simulink model "CtrlStrct_VNT_Level1"  (R2018a)
settings: Solver=VariableStepAuto  StartTime=0.0  StopTime=10  FixedStep=sampletime  RelTol=1e-3  EnableMultiTasking=on
PreLoadFcn:
  | CtrlStrct_SmplCAN_BusInfo
libraries: canmsglib x56, simulink x1
(part 1 of 3)
settings Model: Creator=IAEC nishito  LastModifiedBy=E00026
settings DataIOCC: LimitDataPoints=on  SaveFormat=Array  SaveOutput=off  SaveTime=off
settings OptimizationCC: DefaultParameterBehavior=Inlined  ExpressionDepthLimit=2147483647  LifeSpan=inf
settings DebuggingCC: UnderspecifiedInitializationDetection=Classic  MergeDetectMultiDrivingBlocksExec=none  SolverPrmCheckMsg=warning  InheritedTsInSrcMsg=none  FcnCallInpInsideContextMsg=warning  StateNameClashWarn=warning  SFUnexpectedBacktrackingDiag=warning  SFNoUnconditionalDefaultTransitionDiag=warning  SFExecutionAtInitializationDiag=none
settings HardwareCC: ProdBitPerPointer=32  ProdBitPerSizeT=32  ProdBitPerPtrDiffT=32  ProdLargestAtomicFloat=None  ProdIntDivRoundTo=Undefined  ProdEndianess=Unspecified  ProdWordSize=32  ProdHWDeviceType=32-bit Generic
settings ModelReferenceCC: ModelReferenceNumInstancesAllowed=Single  PropagateSignalLabelsOutOfModel=off
settings CodeAppCC: StateflowObjectComments=on
settings GRTTargetCC: TargetLangStandard=C89/C90 (ANSI)  GeneratePreprocessorConditionals=Disable all  CombineOutputUpdateFcns=off  GRTInterface=on
settings ConfigComp: CovMetricSettings=dw  CovHtmlReporting=on  CovSaveCumulativeToWorkspaceVar=on  CovSaveSingleToWorkspaceVar=on  CovExternalEMLEnable=off

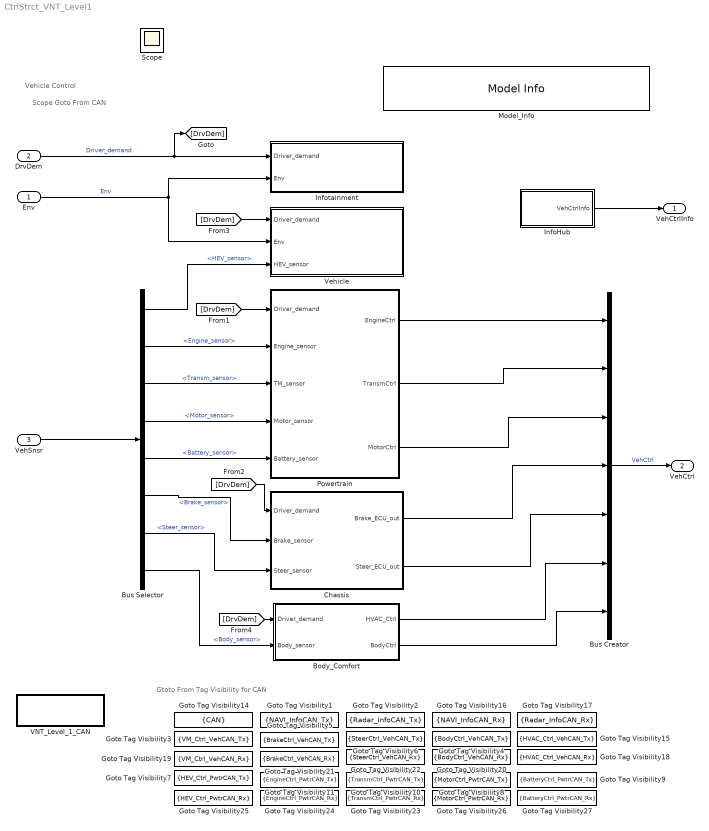
== system CtrlStrct_VNT_Level1 ==
  note: Scope Goto From CAN
  note: Gtoto From Tag Visibility for CAN
  note: Vehicle Control
  Env : Inport  OutDataTypeStr=Bus: Environment_Bus
      settings: AttributesFormatString=<%<OutDataTypeStr>>
  DrvDem : Inport  Port=2  OutDataTypeStr=Bus: Driver_demand_Bus
      settings: AttributesFormatString=%<OutDataTypeStr>
  VehSnsr : Inport  Port=3  OutDataTypeStr=Bus: Vehicle_sensor_Bus
      settings: AttributesFormatString=<%<OutDataTypeStr>>
  Body_Comfort : Subsystem
  Bus Creator : BusCreator  Inputs=7  OutDataTypeStr=Bus: Ctrl_intg_Bus
      settings: AttributesFormatString=%<OutDataTypeStr>
  Bus Selector : BusSelector  OutputSignals=HEV_sensor,Engine_sensor,Transm_sensor,Motor_sensor,Battery_sensor,Brake_sensor,Steer_sensor,Body_sensor
  Chassis : Subsystem
  Goto Tag Visibility1 : GotoTagVisibility  GotoTag=NAVI_InfoCAN_Tx
  Goto Tag Visibility10 : GotoTagVisibility  GotoTag=TransmCtrl_PwtrCAN_Tx
  Goto Tag Visibility11 : GotoTagVisibility  GotoTag=EngineCtrl_PwtrCAN_Tx
  Goto Tag Visibility14 : GotoTagVisibility  GotoTag=CAN
  Goto Tag Visibility15 : GotoTagVisibility  GotoTag=HVAC_Ctrl_VehCAN_Tx
  Goto Tag Visibility16 : GotoTagVisibility  GotoTag=NAVI_InfoCAN_Rx
  Goto Tag Visibility17 : GotoTagVisibility  GotoTag=Radar_InfoCAN_Rx
  Goto Tag Visibility18 : GotoTagVisibility  GotoTag=HVAC_Ctrl_VehCAN_Rx
  Goto Tag Visibility19 : GotoTagVisibility  GotoTag=VM_Ctrl_VehCAN_Rx
  Goto Tag Visibility2 : GotoTagVisibility  GotoTag=Radar_InfoCAN_Tx
  Goto Tag Visibility20 : GotoTagVisibility  GotoTag=BodyCtrl_VehCAN_Rx
  Goto Tag Visibility21 : GotoTagVisibility  GotoTag=BrakeCtrl_VehCAN_Rx
  Goto Tag Visibility22 : GotoTagVisibility  GotoTag=SteerCtrl_VehCAN_Rx
  Goto Tag Visibility23 : GotoTagVisibility  GotoTag=TransmCtrl_PwtrCAN_Rx
  Goto Tag Visibility24 : GotoTagVisibility  GotoTag=EngineCtrl_PwtrCAN_Rx
  Goto Tag Visibility25 : GotoTagVisibility  GotoTag=HEV_Ctrl_PwtrCAN_Rx
  Goto Tag Visibility26 : GotoTagVisibility  GotoTag=MotorCtrl_PwtrCAN_Rx
  Goto Tag Visibility27 : GotoTagVisibility  GotoTag=BatteryCtrl_PwtrCAN_Rx
  Goto Tag Visibility3 : GotoTagVisibility  GotoTag=VM_Ctrl_VehCAN_Tx
  Goto Tag Visibility4 : GotoTagVisibility  GotoTag=BodyCtrl_VehCAN_Tx
  Goto Tag Visibility5 : GotoTagVisibility  GotoTag=BrakeCtrl_VehCAN_Tx
  Goto Tag Visibility6 : GotoTagVisibility  GotoTag=SteerCtrl_VehCAN_Tx
  Goto Tag Visibility7 : GotoTagVisibility  GotoTag=HEV_Ctrl_PwtrCAN_Tx
  Goto Tag Visibility8 : GotoTagVisibility  GotoTag=MotorCtrl_PwtrCAN_Tx
  Goto Tag Visibility9 : GotoTagVisibility  GotoTag=BatteryCtrl_PwtrCAN_Tx
  InfoHub : Subsystem
  Infotainment : Subsystem
  Model_Info : simulink/Model-Wide Utilities/Model Info  Frame=on  DisplayStringWithTags=|  HorizontalTextAlignment=Left  LeftAlignmentValue=0.02
      | Version  %<ModelVersion>
      | LastModifided by %<LastModifiedBy>  Date %<LastModificationDate>
      | Description  %<Description>
  Powertrain : Subsystem
  VNT_Level_1_CAN : Subsystem  VariantControl=VarObj_CanType_VNT_simu
  Vehicle : Subsystem
  VehCtrlInfo : Outport  OutDataTypeStr=Bus: IntgCtrl_Info_Bus
      settings: AttributesFormatString=<%<OutDataTypeStr>>
  VehCtrl : Outport  Port=2  OutDataTypeStr=Bus: Ctrl_intg_Bus
      settings: AttributesFormatString=<%<OutDataTypeStr>>
  Scope : Scope
  wires:
  InfoHub/1(VehCtrlInfo) -> VehCtrlInfo/1
  Chassis/2(Steer_ECU_out) -> Bus Creator/5
  Env/1 -> Vehicle/2(Env), Infotainment/2(Env)  "Env"
  Bus Creator/1 -> VehCtrl/1  "VehCtrl"
  [DrvDem] -> Powertrain/1(Driver_demand)
  Powertrain/3(MotorCtrl) -> Bus Creator/3
  Bus Selector/3 -> Powertrain/3(TM_sensor)  "<Transm_sensor>"
  Bus Selector/6 -> Chassis/2(Brake_sensor)  "<Brake_sensor>"
  Body_Comfort/2(BodyCtrl) -> Bus Creator/7
  Bus Selector/2 -> Powertrain/2(Engine_sensor)  "<Engine_sensor>"
  Powertrain/2(TransmCtrl) -> Bus Creator/2
  Chassis/1(Brake_ECU_out) -> Bus Creator/4
  VehSnsr/1 -> Bus Selector/1
  [DrvDem] -> Chassis/1(Driver_demand)
  Body_Comfort/1(HVAC_Ctrl) -> Bus Creator/6
  Bus Selector/1 -> Vehicle/3(HEV_sensor)  "<HEV_sensor>"
  Bus Selector/7 -> Chassis/3(Steer_sensor)  "<Steer_sensor>"
  Powertrain/1(EngineCtrl) -> Bus Creator/1
  [DrvDem] -> Vehicle/1(Driver_demand)
  Bus Selector/5 -> Powertrain/5(Battery_sensor)  "<Battery_sensor>"
  DrvDem/1 -> [DrvDem], Infotainment/1(Driver_demand)  "Driver_demand"
  Bus Selector/8 -> Body_Comfort/2(Body_sensor)  "<Body_sensor>"
  Bus Selector/4 -> Powertrain/4(Motor_sensor)  "<Motor_sensor>"
  [DrvDem] -> Body_Comfort/1(Driver_demand)

== system CtrlStrct_VNT_Level1/Body_Comfort ==
  note: Body Control
  Driver_demand : Inport
  Body_sensor : Inport  Port=2
  Body_Control : Subsystem
  HVAC_Control : Subsystem
  HVAC_Ctrl : Outport
  BodyCtrl : Outport  Port=2
  wires:
  Body_Control/1(BodyCtrl) -> BodyCtrl/1
  Driver_demand/1 -> HVAC_Control/1(Driver_demand), Body_Control/1(Driver_demand)
  Body_sensor/1 -> HVAC_Control/2(Body_sensor), Body_Control/2(Body_sensor)
  HVAC_Control/1(HVAC_Ctrl) -> HVAC_Ctrl/1

== system CtrlStrct_VNT_Level1/Chassis ==
  note: Chassis Control
  Driver_demand : Inport
  Brake_sensor : Inport  Port=2
  Steer_sensor : Inport  Port=3
  Brake_Control : Subsystem
  Steer_Control : Subsystem
  Brake_ECU_out : Outport
  Steer_ECU_out : Outport  Port=2
  wires:
  Driver_demand/1 -> Brake_Control/1(Driver_demand), Steer_Control/1(Driver_demand)
  Brake_Control/1(BrakeCtrl) -> Brake_ECU_out/1
  Brake_sensor/1 -> Brake_Control/2(Brake_sensor)
  Steer_Control/1(SteerCtrl) -> Steer_ECU_out/1
  Steer_sensor/1 -> Steer_Control/2(Steer_sensor)

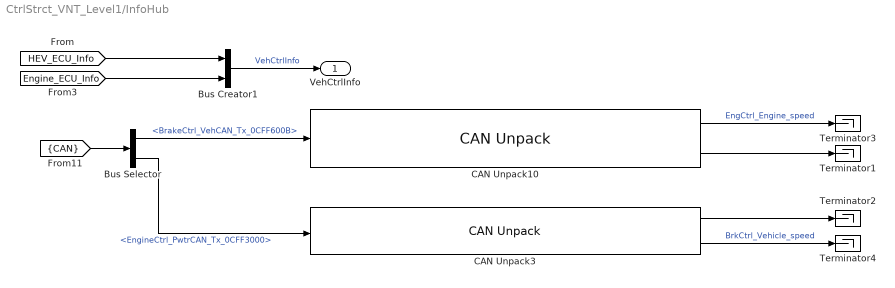
== system CtrlStrct_VNT_Level1/InfoHub ==
  Bus Creator1 : BusCreator  Inputs=2
  Bus Selector : BusSelector  OutputSignals=VehCAN.BrakeCtrl_VehCAN_Tx_0CFF600B,PwtrCAN.EngineCtrl_PwtrCAN_Tx_0CFF3000
  CAN Unpack10 : canmsglib/CAN Unpack  CANdbFile=C:\Users\aa781680\OneDrive - YanmarGlobal\MainStrage\04_MATLAB\JMAAB_CoopCon\CoopConModel\20180726_18a_ymr\Project\CANDB\HEV_CANDB.dbc  MsgList=EngineCtrl_PwtrCAN_Tx  MsgName=EngineCtrl_PwtrCAN_Tx  MsgIDType=Extended (29-bit identifier)  MsgIdentifier=218050560  MsgLength=8  SignalInfo=EngCtrl_Engine_speed$0$16$1$2$1$0$1.250000e-01$0$0$8192$#EngCtrl_Engine_torque_actual$16$16$1$1$1$0$1.562500e-02$0$-300$300$#  NSignals=2  IDPort=off  TimestampPort=off  ErrorPort=off  RemotePort=off  LengthPort=off  StatusPort=off  StartBits=str2num('[int32(0);int32(16)]')  SignalSizes=str2num('[int32(16);int32(16)]')  ByteOrders=str2num('[int32(1);int32(1)]')  DataTypes=str2num('[int32(2);int32(1)]')  MultiplexTypes=str2num('[int32(1);int32(1)]')  MultiplexValues=str2num('[double(0);double(0)]')  Factors=str2num('[double(1.250000e-01);double(1.562500e-02)]')  Offsets=str2num('[double(0);double(0)]')  Minimums=str2num('[double(0);double(-300)]')  Maximums=str2num('[double(8192);double(300)]')  ApplyMinMax=off
      settings: SourceProductName=Simulink Real-Time  SourceProductBaseCode=XP  DataFormat=CANdb specified signals
  CAN Unpack3 : canmsglib/CAN Unpack  CANdbFile=C:\Users\aa781680\OneDrive - YanmarGlobal\MainStrage\04_MATLAB\JMAAB_CoopCon\CoopConModel\20180726_18a_ymr\Project\CANDB\HEV_CANDB.dbc  MsgList=BrakeCtrl_VehCAN_Tx  MsgName=BrakeCtrl_VehCAN_Tx  MsgIDType=Extended (29-bit identifier)  MsgIdentifier=218062859  MsgLength=8  SignalInfo=BrkCtrl_Regen_brake_torque_reque$16$16$1$1$1$0$1.000000e-02$0$-300$300$#BrkCtrl_Vehicle_speed$0$16$1$2$1$0$1.000000e-01$0$0$180$#  NSignals=2  IDPort=off  TimestampPort=off  ErrorPort=off  RemotePort=off  LengthPort=off  StatusPort=off  StartBits=str2num('[int32(16);int32(0)]')  SignalSizes=str2num('[int32(16);int32(16)]')  ByteOrders=str2num('[int32(1);int32(1)]')  DataTypes=str2num('[int32(1);int32(2)]')  MultiplexTypes=str2num('[int32(1);int32(1)]')  MultiplexValues=str2num('[double(0);double(0)]')  Factors=str2num('[double(1.000000e-02);double(1.000000e-01)]')  Offsets=str2num('[double(0);double(0)]')  Minimums=str2num('[double(-300);double(0)]')  Maximums=str2num('[double(300);double(180)]')  ApplyMinMax=off
      settings: SourceProductName=Simulink Real-Time  SourceProductBaseCode=XP  DataFormat=CANdb specified signals
  Terminator{1..4} (4 alike) : Terminator
  VehCtrlInfo : Outport
  wires:
  [CAN] -> Bus Selector/1
  Bus Creator1/1 -> VehCtrlInfo/1  "VehCtrlInfo"
  [Engine_ECU_Info] -> Bus Creator1/2
  [HEV_ECU_Info] -> Bus Creator1/1
  CAN Unpack10/2 -> Terminator1/1
  CAN Unpack3/1 -> Terminator2/1
  Bus Selector/1 -> CAN Unpack10/1  "<BrakeCtrl_VehCAN_Tx_0CFF600B>"
  Bus Selector/2 -> CAN Unpack3/1  "<EngineCtrl_PwtrCAN_Tx_0CFF3000>"
  CAN Unpack10/1 -> Terminator3/1  "EngCtrl_Engine_speed"
  CAN Unpack3/2 -> Terminator4/1  "BrkCtrl_Vehicle_speed"

== system CtrlStrct_VNT_Level1/Infotainment ==
  note: Infotainment
  Driver_demand : Inport
  Env : Inport  Port=2
  Navigation : Subsystem
  Radar_Detection : Subsystem
  wires:
  Env/1 -> Navigation/2(Env), Radar_Detection/2(Env)
  Driver_demand/1 -> Radar_Detection/1(Driver_demand), Navigation/1(Driver_demand)

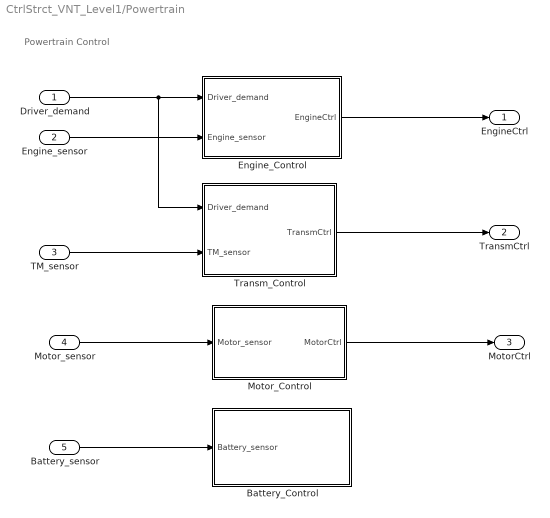
== system CtrlStrct_VNT_Level1/Powertrain ==
  note: Powertrain Control
  Driver_demand : Inport
  Engine_sensor : Inport  Port=2
  TM_sensor : Inport  Port=3
  Motor_sensor : Inport  Port=4
  Battery_sensor : Inport  Port=5
  Battery_Control : Subsystem
  Engine_Control : Subsystem
  Motor_Control : Subsystem
  Transm_Control : Subsystem
  EngineCtrl : Outport
  TransmCtrl : Outport  Port=2
  MotorCtrl : Outport  Port=3
  wires:
  Driver_demand/1 -> Transm_Control/1(Driver_demand), Engine_Control/1(Driver_demand)
  Motor_Control/1(MotorCtrl) -> MotorCtrl/1
  Motor_sensor/1 -> Motor_Control/1(Motor_sensor)
  Battery_sensor/1 -> Battery_Control/1(Battery_sensor)
  Engine_Control/1(EngineCtrl) -> EngineCtrl/1
  Engine_sensor/1 -> Engine_Control/2(Engine_sensor)
  Transm_Control/1(TransmCtrl) -> TransmCtrl/1
  TM_sensor/1 -> Transm_Control/2(TM_sensor)

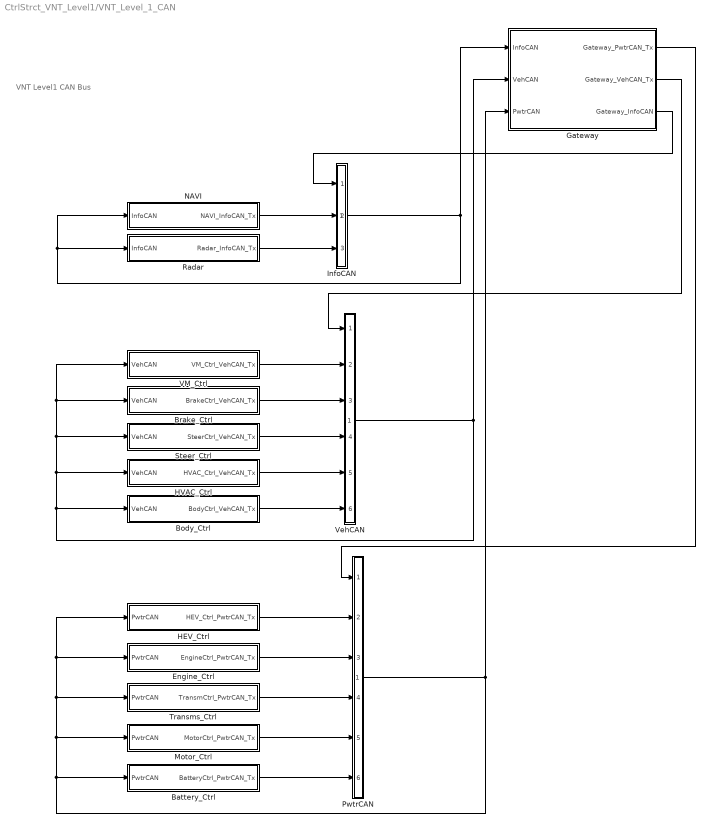
== system CtrlStrct_VNT_Level1/VNT_Level_1_CAN ==
  note: VNT Level1 CAN Bus
  Battery_Ctrl : Subsystem
  Body_Ctrl : Subsystem
  Brake_Ctrl : Subsystem
  Engine_Ctrl : Subsystem
  Gateway : Subsystem
  HEV_Ctrl : Subsystem
  HVAC_Ctrl : Subsystem
  InfoCAN : Subsystem
  Motor_Ctrl : Subsystem
  NAVI : Subsystem
  PwtrCAN : Subsystem
  Radar : Subsystem
  Steer_Ctrl : Subsystem
  Transms_Ctrl : Subsystem
  VM_Ctrl : Subsystem
  VehCAN : Subsystem
  wires:
  PwtrCAN/1(PwtrCAN) -> Battery_Ctrl/1(PwtrCAN), Motor_Ctrl/1(PwtrCAN), Transms_Ctrl/1(PwtrCAN), Engine_Ctrl/1(PwtrCAN), HEV_Ctrl/1(PwtrCAN), Gateway/3(PwtrCAN)
  Gateway/1(Gateway_PwtrCAN_Tx) -> PwtrCAN/1(Gateway_PwtrCAN_Tx)
  HEV_Ctrl/1(HEV_Ctrl_PwtrCAN_Tx) -> PwtrCAN/2(HEV_Ctrl_PwtrCAN_Tx)
  Engine_Ctrl/1(EngineCtrl_PwtrCAN_Tx) -> PwtrCAN/3(EngineCtrl_PwtrCAN_Tx)
  Transms_Ctrl/1(TransmCtrl_PwtrCAN_Tx) -> PwtrCAN/4(TransmCtrl_PwtrCAN_Tx)
  Motor_Ctrl/1(MotorCtrl_PwtrCAN_Tx) -> PwtrCAN/5(MotorCtrl_PwtrCAN_Tx)
  Battery_Ctrl/1(BatteryCtrl_PwtrCAN_Tx) -> PwtrCAN/6(BatteryCtrl_PwtrCAN_Tx)
  VehCAN/1(VehCAN) -> Body_Ctrl/1(VehCAN), HVAC_Ctrl/1(VehCAN), Steer_Ctrl/1(VehCAN), Brake_Ctrl/1(VehCAN), VM_Ctrl/1(VehCAN), Gateway/2(VehCAN)
  Gateway/2(Gateway_VehCAN_Tx) -> VehCAN/1(Gateway_VehCAN_Tx)
  VM_Ctrl/1(VM_Ctrl_VehCAN_Tx) -> VehCAN/2(VM_Ctrl_VehCAN_Tx)
  Brake_Ctrl/1(BrakeCtrl_VehCAN_Tx) -> VehCAN/3(BrakeCtrl_VehCAN_Tx)
  Steer_Ctrl/1(SteerCtrl_VehCAN_Tx) -> VehCAN/4(SteerCtrl_VehCAN_Tx)
  HVAC_Ctrl/1(HVAC_Ctrl_VehCAN_Tx) -> VehCAN/5(HVAC_Ctrl_VehCAN_Tx)
  Body_Ctrl/1(BodyCtrl_VehCAN_Tx) -> VehCAN/6(BodyCtrl_VehCAN_Tx)
  InfoCAN/1(InfoCAN) -> Radar/1(InfoCAN), NAVI/1(InfoCAN), Gateway/1(InfoCAN)
  Gateway/3(Gateway_InfoCAN) -> InfoCAN/1(Gateway_InfoCAN)
  NAVI/1(NAVI_InfoCAN_Tx) -> InfoCAN/2(NAVI_InfoCAN_Tx)
  Radar/1(Radar_InfoCAN_Tx) -> InfoCAN/3(Radar_InfoCAN_Tx)

== system CtrlStrct_VNT_Level1/Vehicle ==
  note: Vehicle Integrated Control
  Driver_demand : Inport
  Env : Inport  Port=2
  HEV_sensor : Inport  Port=3
  HEV_Control : Subsystem
  Vehicle_Motion_Control : Subsystem
  wires:
  Env/1 -> Vehicle_Motion_Control/1(Env)
  Driver_demand/1 -> HEV_Control/1(Driver_demand)
  HEV_sensor/1 -> HEV_Control/2(HEV_sensor)

== system CtrlStrct_VNT_Level1/Body_Comfort/Body_Control ==
  note: Body Control
  Driver_demand : Inport
  Body_sensor : Inport  Port=2
  BodyControlModule : ModelReference  ModelNameDialog=BodyCtrl_V1_1.slx  ModelReferenceVersion=0.1.16
  Rate Transition1 : RateTransition  Deterministic=off
      settings: AttributesFormatString=<Deterministic=%<Deterministic>>
  Rate Transition2 : RateTransition  Deterministic=off
      settings: AttributesFormatString=<Deterministic=%<Deterministic>>
  Rate Transition4 : RateTransition  Deterministic=off
      settings: AttributesFormatString=<Deterministic=%<Deterministic>>
  BodyCtrl : Outport
  tag scope: BodyCtrl_VehCAN_Tx=scoped
  wires:
  Driver_demand/1 -> Rate Transition2/1
  Rate Transition2/1 -> BodyControlModule/1
  BodyControlModule/1 -> Rate Transition4/1
  [BodyCtrl_VehCAN_Rx] -> BodyControlModule/3
  BodyControlModule/2 -> [BodyCtrl_VehCAN_Tx]  "BodyCtrl_VehCAN_Tx"
  Rate Transition4/1 -> BodyCtrl/1  "BodyCtrl"
  Body_sensor/1 -> Rate Transition1/1
  Rate Transition1/1 -> BodyControlModule/2

== system CtrlStrct_VNT_Level1/Body_Comfort/HVAC_Control ==
  note: HVAC Control
  Driver_demand : Inport
  Body_sensor : Inport  Port=2
  Aircon_Control : ModelReference  ModelNameDialog=HVAC_Ctrl_V1_1.slx  ModelReferenceVersion=0.1.25
  Rate Transition1 : RateTransition  Deterministic=off
      settings: AttributesFormatString=<Deterministic=%<Deterministic>>
  Rate Transition2 : RateTransition  Deterministic=off
      settings: AttributesFormatString=<Deterministic=%<Deterministic>>
  Rate Transition4 : RateTransition  Deterministic=off
      settings: AttributesFormatString=<Deterministic=%<Deterministic>>
  HVAC_Ctrl : Outport
  tag scope: HVAC_Ctrl_VehCAN_Tx=scoped
  wires:
  Rate Transition1/1 -> Aircon_Control/2
  Body_sensor/1 -> Rate Transition1/1
  Rate Transition4/1 -> HVAC_Ctrl/1  "HVAC_Ctrl"
  Aircon_Control/2 -> [HVAC_Ctrl_VehCAN_Tx]  "HVAC_Ctrl_VehCAN_Tx"
  [HVAC_Ctrl_VehCAN_Rx] -> Aircon_Control/3
  Aircon_Control/1 -> Rate Transition4/1
  Rate Transition2/1 -> Aircon_Control/1
  Driver_demand/1 -> Rate Transition2/1

== system CtrlStrct_VNT_Level1/Chassis/Brake_Control ==
  note: Brake Control
  Driver_demand : Inport
  Brake_sensor : Inport  Port=2
  Brake_Control : ModelReference  ModelNameDialog=BrakeCtrl_V1_1.slx  ModelReferenceVersion=1.0.23
  Rate Transition1 : RateTransition  Deterministic=off
      settings: AttributesFormatString=<Deterministic=%<Deterministic>>
  Rate Transition2 : RateTransition  Deterministic=off
      settings: AttributesFormatString=<Deterministic=%<Deterministic>>
  Rate Transition4 : RateTransition  Deterministic=off
      settings: AttributesFormatString=<Deterministic=%<Deterministic>>
  Terminator : Terminator
  BrakeCtrl : Outport
  tag scope: BrakeCtrl_VehCAN_Tx=scoped
  wires:
  Rate Transition2/1 -> Brake_Control/2
  Driver_demand/1 -> Rate Transition1/1
  Rate Transition1/1 -> Brake_Control/1
  Brake_sensor/1 -> Rate Transition2/1
  Brake_Control/3 -> Terminator/1
  [BrakeCtrl_VehCAN_Rx] -> Brake_Control/3
  Rate Transition4/1 -> BrakeCtrl/1  "BrakeCtrl"
  Brake_Control/1 -> Rate Transition4/1
  Brake_Control/2 -> [BrakeCtrl_VehCAN_Tx]  "BrakeCtrl_VehCAN_Tx"

== system CtrlStrct_VNT_Level1/Chassis/Steer_Control ==
  note: Steering Control
  Driver_demand : Inport
  Steer_sensor : Inport  Port=2
  Rate Transition3 : RateTransition  Deterministic=off
      settings: AttributesFormatString=<Deterministic=%<Deterministic>>
  Rate Transition4 : RateTransition  Deterministic=off
      settings: AttributesFormatString=<Deterministic=%<Deterministic>>
  Rate Transition5 : RateTransition  Deterministic=off
      settings: AttributesFormatString=<Deterministic=%<Deterministic>>
  Steer_Control : ModelReference  ModelNameDialog=SteerCtrl_V1_1.slx  ModelReferenceVersion=0.1.16
  SteerCtrl : Outport
  tag scope: SteerCtrl_VehCAN_Tx=scoped
  wires:
  Rate Transition4/1 -> Steer_Control/2
  Driver_demand/1 -> Rate Transition3/1
  Steer_Control/1 -> Rate Transition5/1
  Steer_sensor/1 -> Rate Transition4/1
  [SteerCtrl_VehCAN_Rx] -> Steer_Control/3
  Rate Transition3/1 -> Steer_Control/1
  Rate Transition5/1 -> SteerCtrl/1  "SteerCtrl"
  Steer_Control/2 -> [SteerCtrl_VehCAN_Tx]  "SteerCtrl_VehCAN_Tx"

== system CtrlStrct_VNT_Level1/Infotainment/Navigation ==
  note: Navigation
  Driver_demand : Inport
  Env : Inport  Port=2
  NAVI : ModelReference  ModelNameDialog=NAVI_V1_1.slx  ModelReferenceVersion=0.1.17
  Rate Transition1 : RateTransition  Deterministic=off
      settings: AttributesFormatString=<Deterministic=%<Deterministic>>
  Rate Transition4 : RateTransition  Deterministic=off
      settings: AttributesFormatString=<Deterministic=%<Deterministic>>
  tag scope: NAVI_InfoCAN_Tx=scoped
  wires:
  Rate Transition1/1 -> NAVI/1
  Driver_demand/1 -> Rate Transition1/1
  [NAVI_InfoCAN_Rx] -> NAVI/3
  NAVI/1 -> [NAVI_InfoCAN_Tx]  "NAVI_InfoCAN_Tx"
  Env/1 -> Rate Transition4/1
  Rate Transition4/1 -> NAVI/2

== system CtrlStrct_VNT_Level1/Infotainment/Radar_Detection ==
  note: Radar Detection
  Driver_demand : Inport
  Env : Inport  Port=2
  Radar_Detection : ModelReference  ModelNameDialog=Radar_V1_1.slx  ModelReferenceVersion=0.1.17
  Rate Transition1 : RateTransition  Deterministic=off
      settings: AttributesFormatString=<Deterministic=%<Deterministic>>
  Rate Transition4 : RateTransition  Deterministic=off
      settings: AttributesFormatString=<Deterministic=%<Deterministic>>
  tag scope: Radar_InfoCAN_Tx=scoped
  wires:
  Rate Transition1/1 -> Radar_Detection/2
  Env/1 -> Rate Transition1/1
  [Radar_InfoCAN_Rx] -> Radar_Detection/3
  Radar_Detection/1 -> [Radar_InfoCAN_Tx]  "Radar_InfoCAN_Tx"
  Driver_demand/1 -> Rate Transition4/1
  Rate Transition4/1 -> Radar_Detection/1

== system CtrlStrct_VNT_Level1/Powertrain/Battery_Control ==
  note: Battery Control
  Battery_sensor : Inport
  Battery_Control : ModelReference  ModelNameDialog=BatteryCtrl_V1_1.slx  ModelReferenceVersion=0.1.22
  Rate Transition1 : RateTransition  Deterministic=off
      settings: AttributesFormatString=<Deterministic=%<Deterministic>>
  tag scope: BatteryCtrl_PwtrCAN_Tx=scoped
  wires:
  Battery_sensor/1 -> Rate Transition1/1
  [BatteryCtrl_PwtrCAN_Rx] -> Battery_Control/2
  Rate Transition1/1 -> Battery_Control/1
  Battery_Control/1 -> [BatteryCtrl_PwtrCAN_Tx]  "BatteryCtrl_PwtrCAN_Tx"

== system CtrlStrct_VNT_Level1/Powertrain/Engine_Control ==
  note: Engine Control
  Driver_demand : Inport
  Engine_sensor : Inport  Port=2
  Engine_Control : Subsystem  Variant=on
  Info_in : Subsystem
  Rate Transition{1..2,5..6} (4 alike) : RateTransition  Deterministic=off
      settings: AttributesFormatString=<Deterministic=%<Deterministic>>
  EngineCtrl : Outport
  tag scope: EngineCtrl_PwtrCAN_Tx=scoped, Engine_ECU_Info=global
  wires:
  Driver_demand/1 -> Rate Transition1/1
  Engine_sensor/1 -> Rate Transition2/1
  Rate Transition5/1 -> EngineCtrl/1  "EngineCtrl"
  Rate Transition6/1 -> [Engine_ECU_Info]  "EngineCtrl_Info"
  Engine_Control/2(" EngineCtrl_PwtrCAN_Tx") -> [EngineCtrl_PwtrCAN_Tx]  "EngineCtrl_PwtrCAN_Tx"
  Rate Transition1/1 -> Engine_Control/1("DrvDem ")
  Rate Transition2/1 -> Engine_Control/2("Eng_Sns ")
  [EngineCtrl_PwtrCAN_Rx] -> Engine_Control/3(EngineCtrl_PwtrCAN_Rx)
  Info_in/1(Info_in) -> Engine_Control/4("Info_in ")
  Engine_Control/1(" EngineCtrl") -> Rate Transition5/1
  Engine_Control/3(" EngineCtrl_Info") -> Rate Transition6/1

== system CtrlStrct_VNT_Level1/Powertrain/Motor_Control ==
  note: Motor Control
  Motor_sensor : Inport
  Motor_Control : ModelReference  ModelNameDialog=MotorCtrl_V1_1.slx  ModelReferenceVersion=1.0.21
  Rate Transition1 : RateTransition  Deterministic=off
      settings: AttributesFormatString=<Deterministic=%<Deterministic>>
  Rate Transition3 : RateTransition  Deterministic=off
      settings: AttributesFormatString=<Deterministic=%<Deterministic>>
  Terminator : Terminator
  MotorCtrl : Outport
  tag scope: MotorCtrl_PwtrCAN_Tx=scoped
  wires:
  Rate Transition1/1 -> Motor_Control/1
  [MotorCtrl_PwtrCAN_Rx] -> Motor_Control/2
  Motor_sensor/1 -> Rate Transition1/1
  Motor_Control/3 -> Terminator/1
  Rate Transition3/1 -> MotorCtrl/1  "MotorCtrl"
  Motor_Control/1 -> Rate Transition3/1
  Motor_Control/2 -> [MotorCtrl_PwtrCAN_Tx]  "MotorCtrl_PwtrCAN_Tx"

== system CtrlStrct_VNT_Level1/Powertrain/Transm_Control ==
  note: Transmission Control
  Driver_demand : Inport
  TM_sensor : Inport  Port=2
  Rate Transition3 : RateTransition  Deterministic=off
      settings: AttributesFormatString=<Deterministic=%<Deterministic>>
  Rate Transition4 : RateTransition  Deterministic=off
      settings: AttributesFormatString=<Deterministic=%<Deterministic>>
  Rate Transition5 : RateTransition  Deterministic=off
      settings: AttributesFormatString=<Deterministic=%<Deterministic>>
  Terminator : Terminator
  Transm_ECU : ModelReference  ModelNameDialog=TransmCtrl_V1_1.slx  ModelReferenceVersion=1.0.41
  TransmCtrl : Outport
  tag scope: TransmCtrl_PwtrCAN_Tx=scoped
  wires:
  Rate Transition4/1 -> Transm_ECU/2
  Transm_ECU/3 -> Terminator/1
  Driver_demand/1 -> Rate Transition3/1
  TM_sensor/1 -> Rate Transition4/1
  [TransmCtrl_PwtrCAN_Rx] -> Transm_ECU/3
  Rate Transition3/1 -> Transm_ECU/1
  Rate Transition5/1 -> TransmCtrl/1  "TransmCtrl"
  Transm_ECU/1 -> Rate Transition5/1
  Transm_ECU/2 -> [TransmCtrl_PwtrCAN_Tx]  "TransmCtrl_PwtrCAN_Tx"

== system CtrlStrct_VNT_Level1/VNT_Level_1_CAN/Battery_Ctrl ==
  note: Battery control
  note: CAN receive and transmit
  note: Battery Control
  PwtrCAN : Inport
  BatteryCtrl_PwtrCAN Tx : Subsystem
  BatteryCtrl_PwtrCAN_Rx : Subsystem
  BatteryCtrl_PwtrCAN_Tx : Outport
  tag scope: BatteryCtrl_PwtrCAN_Rx=scoped
  wires:
  [BatteryCtrl_PwtrCAN_Tx] -> BatteryCtrl_PwtrCAN Tx/1(BatteryCtrl_PwtrCAN_Tx_Apli)
  BatteryCtrl_PwtrCAN Tx/1(BatteryCtrl_PwtrCAN_Tx) -> BatteryCtrl_PwtrCAN_Tx/1
  PwtrCAN/1 -> BatteryCtrl_PwtrCAN_Rx/1(PwtrCAN)
  BatteryCtrl_PwtrCAN_Rx/1(BatteryCtrl_PwtrCAN_Rx) -> [BatteryCtrl_PwtrCAN_Rx]

== system CtrlStrct_VNT_Level1/VNT_Level_1_CAN/Body_Ctrl ==
  note: Body Control
  note: CAN receive and transmit
  note: Body control
  VehCAN : Inport
  BodyCtrl_VehCAN Tx : Subsystem
  BodyCtrl_VehCAN_Rx : Subsystem
  BodyCtrl_VehCAN_Tx : Outport
  tag scope: BodyCtrl_VehCAN_Rx=scoped
  wires:
  [BodyCtrl_VehCAN_Tx] -> BodyCtrl_VehCAN Tx/1(BodyCtrl_VehCAN_Tx_Apli)
  BodyCtrl_VehCAN Tx/1(BodyCtrl_VehCAN_Tx) -> BodyCtrl_VehCAN_Tx/1
  VehCAN/1 -> BodyCtrl_VehCAN_Rx/1(VehCAN)
  BodyCtrl_VehCAN_Rx/1(BodyCtrl_VehCAN_Rx) -> [BodyCtrl_VehCAN_Rx]

== system CtrlStrct_VNT_Level1/VNT_Level_1_CAN/Brake_Ctrl ==
  note: Brake Control
  note: CAN receive and transmit
  note: Brake control
  VehCAN : Inport
  BrakeCtrl_VehCAN Tx : Subsystem
  BrakeCtrl_VehCAN_Rx : Subsystem
  BrakeCtrl_VehCAN_Tx : Outport
  tag scope: BrakeCtrl_VehCAN_Rx=scoped
  wires:
  [BrakeCtrl_VehCAN_Tx] -> BrakeCtrl_VehCAN Tx/1(BrakeCtrl_VehCAN_Tx_Apli)
  BrakeCtrl_VehCAN Tx/1(BrakeCtrl_VehCAN_Tx) -> BrakeCtrl_VehCAN_Tx/1
  VehCAN/1 -> BrakeCtrl_VehCAN_Rx/1(VehCAN)
  BrakeCtrl_VehCAN_Rx/1(BrakeCtrl_VehCAN_Rx) -> [BrakeCtrl_VehCAN_Rx]

== system CtrlStrct_VNT_Level1/VNT_Level_1_CAN/Engine_Ctrl ==
  note: Engine control
  note: Engine Control
  note: CAN receive and transmit
  PwtrCAN : Inport
  EngineCtrl_PwtrCAN Tx : Subsystem
  EngineCtrl_PwtrCAN_Rx : Subsystem
  EngineCtrl_PwtrCAN_Tx : Outport
  tag scope: EngineCtrl_PwtrCAN_Rx=scoped
  wires:
  [EngineCtrl_PwtrCAN_Tx] -> EngineCtrl_PwtrCAN Tx/1(EngineCtrl_PwtrCAN_Tx_Apli)
  EngineCtrl_PwtrCAN Tx/1(EngineCtrl_PwtrCAN_Tx) -> EngineCtrl_PwtrCAN_Tx/1
  PwtrCAN/1 -> EngineCtrl_PwtrCAN_Rx/1(PwtrCAN)
  EngineCtrl_PwtrCAN_Rx/1(EngineCtrl_PwtrCAN_Rx) -> [EngineCtrl_PwtrCAN_Rx]

== system CtrlStrct_VNT_Level1/VNT_Level_1_CAN/Gateway ==
  note: Gateway
  InfoCAN : Inport
  VehCAN : Inport  Port=2
  PwtrCAN : Inport  Port=3
  Gateway InfoCAN : Subsystem
  Gateway PwtrCAN : Subsystem
  Gateway VehCAN : Subsystem
  Info Hub : Subsystem
  Gateway_PwtrCAN_Tx : Outport
  Gateway_VehCAN_Tx : Outport  Port=2
  Gateway_InfoCAN : Outport  Port=3
  wires:
  InfoCAN/1 -> Info Hub/1(InfoCAN), Gateway PwtrCAN/1(InfoCAN), Gateway VehCAN/1(InfoCAN)
  VehCAN/1 -> Info Hub/2(VehCAN), Gateway PwtrCAN/2(VehCAN), Gateway InfoCAN/1(VehCAN)
  PwtrCAN/1 -> Info Hub/3(PwtrCAN), Gateway VehCAN/2(PwtrCAN)
  Gateway InfoCAN/1(Gateway_InfoCAN) -> Gateway_InfoCAN/1
  Gateway VehCAN/1(Gateway_VehCAN_Tx) -> Gateway_VehCAN_Tx/1
  Gateway PwtrCAN/1(Gateway_PwtrCAN_Tx) -> Gateway_PwtrCAN_Tx/1

== system CtrlStrct_VNT_Level1/VNT_Level_1_CAN/HEV_Ctrl ==
  note: HEV control
  note: HEV control
  note: CAN receive and transmit
  PwtrCAN : Inport
  HEV_Ctrl_PwtrCAN Tx : Subsystem
  HEV_Ctrl_PwtrCAN_Rx : Subsystem
  HEV_Ctrl_PwtrCAN_Tx : Outport
  tag scope: HEV_Ctrl_PwtrCAN_Rx=scoped
  wires:
  [HEV_Ctrl_PwtrCAN_Tx] -> HEV_Ctrl_PwtrCAN Tx/1(HEV_Ctrl_PwtrCAN_Tx_Apli)
  HEV_Ctrl_PwtrCAN Tx/1(HEV_Ctrl_PwtrCAN_Tx) -> HEV_Ctrl_PwtrCAN_Tx/1
  PwtrCAN/1 -> HEV_Ctrl_PwtrCAN_Rx/1(PwtrCAN)
  HEV_Ctrl_PwtrCAN_Rx/1(HEV_Ctrl_PwtrCAN_Rx) -> [HEV_Ctrl_PwtrCAN_Rx]

== system CtrlStrct_VNT_Level1/VNT_Level_1_CAN/HVAC_Ctrl ==
  note: HVAC control
  note: CAN receive and transmit
  note: HVAC Control
  VehCAN : Inport
  HVAC_Ctrl_VehCAN Tx : Subsystem
  HVAC_Ctrl_VehCAN_Rx : Subsystem
  HVAC_Ctrl_VehCAN_Tx : Outport
  tag scope: HVAC_Ctrl_VehCAN_Rx=scoped
  wires:
  [HVAC_Ctrl_VehCAN_Tx] -> HVAC_Ctrl_VehCAN Tx/1(HVAC_Ctrl_VehCAN_Tx_Apli)
  HVAC_Ctrl_VehCAN Tx/1(HVAC_Ctrl_VehCAN_Tx) -> HVAC_Ctrl_VehCAN_Tx/1
  VehCAN/1 -> HVAC_Ctrl_VehCAN_Rx/1(VehCAN)
  HVAC_Ctrl_VehCAN_Rx/1(HVAC_Ctrl_VehCAN_Rx) -> [HVAC_Ctrl_VehCAN_Rx]

== system CtrlStrct_VNT_Level1/VNT_Level_1_CAN/InfoCAN ==
  Gateway_InfoCAN : Inport
  NAVI_InfoCAN_Tx : Inport  Port=2
  Radar_InfoCAN_Tx : Inport  Port=3
  Bus Creator : BusCreator  Inputs=3
  Bus Selector : BusSelector  OutputSignals=Gateway_InfoCAN_Tx_0CFFC485
  Bus Selector1 : BusSelector  OutputSignals=NAVI_InfoCAN_Tx_0CFFB01C
  Bus Selector2 : BusSelector  OutputSignals=Radar_InfoCAN_Tx_0CFF0080
  CAN_Memory : Memory
  InfoCAN : Outport
  wires:
  Bus Creator/1 -> CAN_Memory/1  "InfoCAN"
  Radar_InfoCAN_Tx/1 -> Bus Selector2/1
  CAN_Memory/1 -> InfoCAN/1  "InfoCAN"
  Gateway_InfoCAN/1 -> Bus Selector/1
  NAVI_InfoCAN_Tx/1 -> Bus Selector1/1
  Bus Selector/1 -> Bus Creator/1  "<Gateway_InfoCAN_Tx_0CFFC485>"
  Bus Selector1/1 -> Bus Creator/2  "<NAVI_InfoCAN_Tx_0CFFB01C>"
  Bus Selector2/1 -> Bus Creator/3  "<Radar_InfoCAN_Tx_0CFF0080>"

== system CtrlStrct_VNT_Level1/VNT_Level_1_CAN/Motor_Ctrl ==
  note: Motor control
  note: Motor Control
  note: CAN receive and transmit
  PwtrCAN : Inport
  MotorCtrl_PwtrCAN Tx : Subsystem
  MotorCtrl_PwtrCAN_Rx : Subsystem
  MotorCtrl_PwtrCAN_Tx : Outport
  tag scope: MotorCtrl_PwtrCAN_Rx=scoped
  wires:
  [MotorCtrl_PwtrCAN_Tx] -> MotorCtrl_PwtrCAN Tx/1(IMotorCtrl_PwtrCAN_Tx_Apli)
  MotorCtrl_PwtrCAN Tx/1(MotorCtrl_PwtrCAN_Tx_0CFF5083) -> MotorCtrl_PwtrCAN_Tx/1
  PwtrCAN/1 -> MotorCtrl_PwtrCAN_Rx/1(PwtrCAN)
  MotorCtrl_PwtrCAN_Rx/1(MotorCtrl_PwtrCAN_Rx) -> [MotorCtrl_PwtrCAN_Rx]

== system CtrlStrct_VNT_Level1/VNT_Level_1_CAN/NAVI ==
  note: Navigation
  note: CAN receive and transmit
  note: Navigation
  InfoCAN : Inport
  NAVI_InfoCAN Tx : Subsystem
  NAVI_InfoCAN_Rx : Subsystem
  NAVI_InfoCAN_Tx : Outport
  tag scope: NAVI_InfoCAN_Rx=scoped
  wires:
  [NAVI_InfoCAN_Tx] -> NAVI_InfoCAN Tx/1(NAVI_InfoCAN_Tx_Apli)
  NAVI_InfoCAN_Rx/1(NAVI_InfoCAN_Rx) -> [NAVI_InfoCAN_Rx]
  InfoCAN/1 -> NAVI_InfoCAN_Rx/1(InfoCAN)
  NAVI_InfoCAN Tx/1(NAVI_InfoCAN_Tx) -> NAVI_InfoCAN_Tx/1

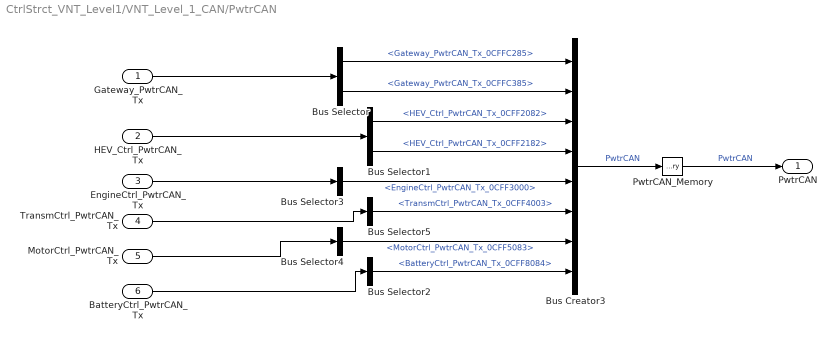
== system CtrlStrct_VNT_Level1/VNT_Level_1_CAN/PwtrCAN ==
  Gateway_PwtrCAN_Tx : Inport
  HEV_Ctrl_PwtrCAN_Tx : Inport  Port=2
  EngineCtrl_PwtrCAN_Tx : Inport  Port=3
  TransmCtrl_PwtrCAN_Tx : Inport  Port=4
  MotorCtrl_PwtrCAN_Tx : Inport  Port=5
  BatteryCtrl_PwtrCAN_Tx : Inport  Port=6
  Bus Creator3 : BusCreator  Inputs=8
  Bus Selector : BusSelector  OutputSignals=Gateway_PwtrCAN_Tx_0CFFC285,Gateway_PwtrCAN_Tx_0CFFC385
  Bus Selector1 : BusSelector  OutputSignals=HEV_Ctrl_PwtrCAN_Tx_0CFF2082,HEV_Ctrl_PwtrCAN_Tx_0CFF2182
  Bus Selector2 : BusSelector  OutputSignals=BatteryCtrl_PwtrCAN_Tx_0CFF8084
  Bus Selector3 : BusSelector  OutputSignals=EngineCtrl_PwtrCAN_Tx_0CFF3000
  Bus Selector4 : BusSelector  OutputSignals=MotorCtrl_PwtrCAN_Tx_0CFF5083
  Bus Selector5 : BusSelector  OutputSignals=TransmCtrl_PwtrCAN_Tx_0CFF4003
  PwtrCAN_Memory : Memory
  PwtrCAN : Outport
  wires:
  TransmCtrl_PwtrCAN_Tx/1 -> Bus Selector5/1
  Bus Creator3/1 -> PwtrCAN_Memory/1  "PwtrCAN"
  EngineCtrl_PwtrCAN_Tx/1 -> Bus Selector3/1
  Gateway_PwtrCAN_Tx/1 -> Bus Selector/1
  HEV_Ctrl_PwtrCAN_Tx/1 -> Bus Selector1/1
  BatteryCtrl_PwtrCAN_Tx/1 -> Bus Selector2/1
  MotorCtrl_PwtrCAN_Tx/1 -> Bus Selector4/1
  PwtrCAN_Memory/1 -> PwtrCAN/1  "PwtrCAN"
  Bus Selector/1 -> Bus Creator3/1  "<Gateway_PwtrCAN_Tx_0CFFC285>"
  Bus Selector/2 -> Bus Creator3/2  "<Gateway_PwtrCAN_Tx_0CFFC385>"
  Bus Selector1/1 -> Bus Creator3/3  "<HEV_Ctrl_PwtrCAN_Tx_0CFF2082>"
  Bus Selector1/2 -> Bus Creator3/4  "<HEV_Ctrl_PwtrCAN_Tx_0CFF2182>"
  Bus Selector2/1 -> Bus Creator3/8  "<BatteryCtrl_PwtrCAN_Tx_0CFF8084>"
  Bus Selector3/1 -> Bus Creator3/5  "<EngineCtrl_PwtrCAN_Tx_0CFF3000>"
  Bus Selector4/1 -> Bus Creator3/7  "<MotorCtrl_PwtrCAN_Tx_0CFF5083>"
  Bus Selector5/1 -> Bus Creator3/6  "<TransmCtrl_PwtrCAN_Tx_0CFF4003>"

== system CtrlStrct_VNT_Level1/VNT_Level_1_CAN/Radar ==
  note: Radar detection
  note: CAN receive and transmit
  note: Radar Detection
  InfoCAN : Inport
  Radar_InfoCAN Tx : Subsystem
  Radar_InfoCAN_Rx : Subsystem
  Radar_InfoCAN_Tx : Outport
  tag scope: Radar_InfoCAN_Rx=scoped
  wires:
  Radar_InfoCAN_Rx/1(Radar_InfoCAN_Rx) -> [Radar_InfoCAN_Rx]
  InfoCAN/1 -> Radar_InfoCAN_Rx/1(InfoCAN)
  [Radar_InfoCAN_Tx] -> Radar_InfoCAN Tx/1(Radar_InfoCAN_Tx_Apli)
  Radar_InfoCAN Tx/1(Radar_InfoCAN_Tx) -> Radar_InfoCAN_Tx/1

== system CtrlStrct_VNT_Level1/VNT_Level_1_CAN/Steer_Ctrl ==
  note: Steering control
  note: CAN receive and transmit
  note: Steering Control
  VehCAN : Inport
  SteerCtrl_VehCAN Tx : Subsystem
  SteerCtrl_VehCAN_Rx : Subsystem
  SteerCtrl_VehCAN_Tx : Outport
  tag scope: SteerCtrl_VehCAN_Rx=scoped
  wires:
  [SteerCtrl_VehCAN_Tx] -> SteerCtrl_VehCAN Tx/1(SteerCtrl_VehCAN_Tx_Apli)
  SteerCtrl_VehCAN Tx/1(SteerCtrl_VehCAN_Tx) -> SteerCtrl_VehCAN_Tx/1
  VehCAN/1 -> SteerCtrl_VehCAN_Rx/1(VehCAN)
  SteerCtrl_VehCAN_Rx/1(SteerCtrl_VehCAN_Rx) -> [SteerCtrl_VehCAN_Rx]

== system CtrlStrct_VNT_Level1/VNT_Level_1_CAN/Transms_Ctrl ==
  note: Transmission control
  note: CAN receive and transmit
  note: Transmission Control
  PwtrCAN : Inport
  TransmCtrl_PwtrCAN Tx : Subsystem
  TransmCtrl_PwtrCAN_Rx : Subsystem
  TransmCtrl_PwtrCAN_Tx : Outport
  tag scope: TransmCtrl_PwtrCAN_Rx=scoped
  wires:
  [TransmCtrl_PwtrCAN_Tx] -> TransmCtrl_PwtrCAN Tx/1(TransmCtrl_PwtrCAN_Tx_Apli)
  TransmCtrl_PwtrCAN Tx/1(TransmCtrl_PwtrCAN_Tx) -> TransmCtrl_PwtrCAN_Tx/1
  PwtrCAN/1 -> TransmCtrl_PwtrCAN_Rx/1(PwtrCAN)
  TransmCtrl_PwtrCAN_Rx/1(TransmCtrl_PwtrCAN_Rx) -> [TransmCtrl_PwtrCAN_Rx]

== system CtrlStrct_VNT_Level1/VNT_Level_1_CAN/VM_Ctrl ==
  note: Vehicle motion control
  note: Vehicle Motion Control
  note: CAN receive and transmit
  VehCAN : Inport
  VM_Ctrl_VehCAN Tx : Subsystem
  VM_Ctrl_VehCAN_Rx : Subsystem
  VM_Ctrl_VehCAN_Tx : Outport
  tag scope: VM_Ctrl_VehCAN_Rx=scoped
  wires:
  [VM_Ctrl_VehCAN_Tx] -> VM_Ctrl_VehCAN Tx/1(VM_Ctrl_VehCAN_Tx_Apli)
  VM_Ctrl_VehCAN Tx/1(VM_Ctrl_VehCAN_Tx) -> VM_Ctrl_VehCAN_Tx/1
  VehCAN/1 -> VM_Ctrl_VehCAN_Rx/1(VehCAN)
  VM_Ctrl_VehCAN_Rx/1(VM_Ctrl_VehCAN_Rx) -> [VM_Ctrl_VehCAN_Rx]

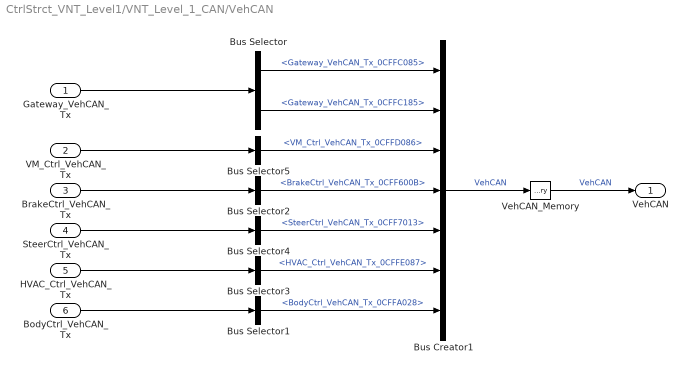
== system CtrlStrct_VNT_Level1/VNT_Level_1_CAN/VehCAN ==
  Gateway_VehCAN_Tx : Inport
  VM_Ctrl_VehCAN_Tx : Inport  Port=2
  BrakeCtrl_VehCAN_Tx : Inport  Port=3
  SteerCtrl_VehCAN_Tx : Inport  Port=4
  HVAC_Ctrl_VehCAN_Tx : Inport  Port=5
  BodyCtrl_VehCAN_Tx : Inport  Port=6
  Bus Creator1 : BusCreator  Inputs=7
  Bus Selector : BusSelector  OutputSignals=Gateway_VehCAN_Tx_0CFFC085,Gateway_VehCAN_Tx_0CFFC185
  Bus Selector1 : BusSelector  OutputSignals=BodyCtrl_VehCAN_Tx_0CFFA028
  Bus Selector2 : BusSelector  OutputSignals=BrakeCtrl_VehCAN_Tx_0CFF600B
  Bus Selector3 : BusSelector  OutputSignals=HVAC_Ctrl_VehCAN_Tx_0CFFE087
  Bus Selector4 : BusSelector  OutputSignals=SteerCtrl_VehCAN_Tx_0CFF7013
  Bus Selector5 : BusSelector  OutputSignals=VM_Ctrl_VehCAN_Tx_0CFFD086
  VehCAN_Memory : Memory
  VehCAN : Outport
  wires:
  VehCAN_Memory/1 -> VehCAN/1  "VehCAN"
  SteerCtrl_VehCAN_Tx/1 -> Bus Selector4/1
  BrakeCtrl_VehCAN_Tx/1 -> Bus Selector2/1
  Gateway_VehCAN_Tx/1 -> Bus Selector/1
  Bus Creator1/1 -> VehCAN_Memory/1  "VehCAN"
  BodyCtrl_VehCAN_Tx/1 -> Bus Selector1/1
  HVAC_Ctrl_VehCAN_Tx/1 -> Bus Selector3/1
  VM_Ctrl_VehCAN_Tx/1 -> Bus Selector5/1
  Bus Selector/1 -> Bus Creator1/1  "<Gateway_VehCAN_Tx_0CFFC085>"
  Bus Selector/2 -> Bus Creator1/2  "<Gateway_VehCAN_Tx_0CFFC185>"
  Bus Selector1/1 -> Bus Creator1/7  "<BodyCtrl_VehCAN_Tx_0CFFA028>"
  Bus Selector2/1 -> Bus Creator1/4  "<BrakeCtrl_VehCAN_Tx_0CFF600B>"
  Bus Selector3/1 -> Bus Creator1/6  "<HVAC_Ctrl_VehCAN_Tx_0CFFE087>"
  Bus Selector4/1 -> Bus Creator1/5  "<SteerCtrl_VehCAN_Tx_0CFF7013>"
  Bus Selector5/1 -> Bus Creator1/3  "<VM_Ctrl_VehCAN_Tx_0CFFD086>"

== system CtrlStrct_VNT_Level1/Vehicle/HEV_Control ==
  note: HEV Control
  Driver_demand : Inport
  HEV_sensor : Inport  Port=2
  HEV_Control : ModelReference  ModelNameDialog=HEV_Ctrl_V1_1.slx  SimulationMode=Normal  ModelReferenceVersion=1.0.50
  Rate Transition2 : RateTransition  Deterministic=off
      settings: AttributesFormatString=<Deterministic=%<Deterministic>>
  Rate Transition3 : RateTransition  Deterministic=off
      settings: AttributesFormatString=<Deterministic=%<Deterministic>>
  Rate Transition4 : RateTransition  Deterministic=off
      settings: AttributesFormatString=<Deterministic=%<Deterministic>>
  tag scope: HEV_Ctrl_PwtrCAN_Tx=scoped, HEV_ECU_Info=global
  wires:
  Driver_demand/1 -> Rate Transition3/1
  [HEV_Ctrl_PwtrCAN_Rx] -> HEV_Control/3
  HEV_sensor/1 -> Rate Transition2/1
  Rate Transition2/1 -> HEV_Control/2
  HEV_Control/2 -> Rate Transition4/1
  Rate Transition4/1 -> [HEV_ECU_Info]  "HEV_Ctrl_Info"
  HEV_Control/1 -> [HEV_Ctrl_PwtrCAN_Tx]  "HEV_Ctrl_PwtrCAN_Tx"
  Rate Transition3/1 -> HEV_Control/1

== system CtrlStrct_VNT_Level1/Vehicle/Vehicle_Motion_Control ==
  note: Vehicle Motion Control
  Env : Inport
  Rate Transition1 : RateTransition  Deterministic=off
      settings: AttributesFormatString=<Deterministic=%<Deterministic>>
  Vehicle_Motion_Control : ModelReference  ModelNameDialog=VM_Ctrl_V1_1.slx  SimulationMode=Normal  ModelReferenceVersion=0.1.26
  tag scope: VM_Ctrl_VehCAN_Tx=scoped
  wires:
  Vehicle_Motion_Control/1 -> [VM_Ctrl_VehCAN_Tx]  "VM_Ctrl_VehCAN_Tx"
  Rate Transition1/1 -> Vehicle_Motion_Control/1
  Env/1 -> Rate Transition1/1
  [VM_Ctrl_VehCAN_Rx] -> Vehicle_Motion_Control/2

== system CtrlStrct_VNT_Level1/Powertrain/Engine_Control/Engine_Control ==
  "DrvDem " : Inport
  "Eng_Sns " : Inport  Port=2
  EngineCtrl_PwtrCAN_Rx : Inport  Port=3
  "Info_in " : Inport  Port=4
  EngineCtrl_V1.slx : ModelReference  ModelNameDialog=EngineCtrl_V1_1.slx  VariantControl=VarObj_EngEcu_Simple  ModelReferenceVersion=1.0.22
  EngineCtrl_V2.slx : ModelReference  ModelNameDialog=EngineCtrl_V2.slx  SimulationMode=Normal  VariantControl=VarObj_EngEcu_Medium  ModelReferenceVersion=1.0.8
  " EngineCtrl" : Outport
  " EngineCtrl_PwtrCAN_Tx" : Outport  Port=2
  " EngineCtrl_Info" : Outport  Port=3

== system CtrlStrct_VNT_Level1/Powertrain/Engine_Control/Info_in ==
  Bus Creator1 : BusCreator  Inputs=1
  Constant : Constant
  Info_in : Outport
  wires:
  Constant/1 -> Bus Creator1/1  "dummy"
  Bus Creator1/1 -> Info_in/1  "Info_in"

== system CtrlStrct_VNT_Level1/VNT_Level_1_CAN/Battery_Ctrl/BatteryCtrl_PwtrCAN Tx ==
  note: Function of CAN transmit
      | ・conversion fromCAN application signal to signal of CAN message
  note: Battery Control
  note: CAN transmit
  BatteryCtrl_PwtrCAN_Tx_Apli : Inport
  BatteryCtrl_PwtrCAN Pack : canmsglib/CAN Pack  CANdbFile=HEV_CANDB.dbc  MsgList=BatteryCtrl_PwtrCAN_Tx  MsgName=BatteryCtrl_PwtrCAN_Tx  MsgIDType=Extended (29-bit identifier)  MsgIdentifier=218071172  MsgLength=8  SignalInfo=BatCtrl_SOC$0$16$1$2$1$0$3.906250e-03$0$0$100$#  NSignals=1  StartBits=str2num('[int32(0)]')  SignalSizes=str2num('[int32(16)]')  ByteOrders=str2num('[int32(1)]')  DataTypes=str2num('[int32(2)]')  MultiplexTypes=str2num('[int32(1)]')  MultiplexValues=str2num('[double(0)]')  Factors=str2num('[double(3.906250e-03)]')  Offsets=str2num('[double(0)]')  Minimums=str2num('[double(0)]')  Maximums=str2num('[double(100)]')  Remote=off  ApplyMinMax=off  BusOutput=off
      settings: AttributesFormatString=<CANdbFile = %<CANdbFile>>  SourceProductName=Simulink Real-Time  SourceProductBaseCode=XP  DataFormat=CANdb specified signals
  Bus Creator1 : BusCreator  Inputs=1
  Bus Selector1 : BusSelector  OutputSignals=BatCtrl_SOC
  BatteryCtrl_PwtrCAN_Tx : Outport
  wires:
  BatteryCtrl_PwtrCAN Pack/1 -> Bus Creator1/1  "BatteryCtrl_PwtrCAN_Tx_0CFF8084"
  Bus Creator1/1 -> BatteryCtrl_PwtrCAN_Tx/1  "BatteryCtrl_PwtrCAN_Tx"
  Bus Selector1/1 -> BatteryCtrl_PwtrCAN Pack/1  "<BatCtrl_SOC>"
  BatteryCtrl_PwtrCAN_Tx_Apli/1 -> Bus Selector1/1

== system CtrlStrct_VNT_Level1/VNT_Level_1_CAN/Battery_Ctrl/BatteryCtrl_PwtrCAN_Rx ==
  note: Function of CAN receive
      | ・CAN message selection
      | ・conversion from CAN signal to CAN application signal with bus object
  note: Battery Control
  note: CAN receive
  PwtrCAN : Inport
  BatteryCtrl_PwtrCAN Unpack : canmsglib/CAN Unpack  CANdbFile=HEV_CANDB.dbc  MsgList=HEV_Ctrl_PwtrCAN_Tx_1  MsgName=HEV_Ctrl_PwtrCAN_Tx_1  MsgIDType=Extended (29-bit identifier)  MsgIdentifier=218046594  MsgLength=8  SignalInfo=HEVCtrl_Engine_torque_request$0$16$1$1$1$0$1.562500e-02$0$-300$300$#HEVCtrl_Motor_torque_request$16$16$1$1$1$0$1.562500e-02$0$-300$300$#HEVCtrl_Regen_brake_torque_actua$48$16$1$1$1$0$6.250000e-02$0$-300$3000$#HEVCtrl_Regen_brake_torque_avail$32$16$1$1$1$0$6.250000e-02$0$-300$3000$#  NSignals=4  IDPort=off  TimestampPort=off  ErrorPort=off  RemotePort=off  LengthPort=off  StatusPort=off  StartBits=str2num('[int32(0);int32(16);int32(48);int32(32)]')  SignalSizes=str2num('[int32(16);int32(16);int32(16);int32(16)]')  ByteOrders=str2num('[int32(1);int32(1);int32(1);int32(1)]')  DataTypes=str2num('[int32(1);int32(1);int32(1);int32(1)]')  MultiplexTypes=str2num('[int32(1);int32(1);int32(1);int32(1)]')  MultiplexValues=str2num('[double(0);double(0);double(0);double(0)]')  Factors=str2num('[double(1.562500e-02);double(1.562500e-02);double(6.250000e-02);double(6.250000e-02)]')  Offsets=str2num('[double(0);double(0);double(0);double(0)]')  Minimums=str2num('[double(-300);double(-300);double(-300);double(-300)]')  Maximums=str2num('[double(300);double(300);double(3000);double(3000)]')  ApplyMinMax=off
      settings: AttributesFormatString=<CANdbFile = %<CANdbFile>>  SourceProductName=Simulink Real-Time  SourceProductBaseCode=XP  DataFormat=CANdb specified signals
  Bus Creator5 : BusCreator  Inputs=1
  Bus Selector2 : BusSelector  OutputSignals=HEV_Ctrl_PwtrCAN_Tx_0CFF2082
  Rate Transition1 : RateTransition  Deterministic=off
      settings: AttributesFormatString=<Deterministic=%<Deterministic>>
  Terminator1 : Terminator
  Terminator2 : Terminator
  Terminator3 : Terminator
  BatteryCtrl_PwtrCAN_Rx : Outport
  wires:
  Bus Creator5/1 -> Rate Transition1/1
  BatteryCtrl_PwtrCAN Unpack/3 -> Terminator2/1
  BatteryCtrl_PwtrCAN Unpack/4 -> Terminator3/1
  BatteryCtrl_PwtrCAN Unpack/2 -> Bus Creator5/1  "HEVCtrl_Motor_torque_request"
  Rate Transition1/1 -> BatteryCtrl_PwtrCAN_Rx/1  "BatteryCtrl_PwtrCAN_Rx"
  BatteryCtrl_PwtrCAN Unpack/1 -> Terminator1/1
  Bus Selector2/1 -> BatteryCtrl_PwtrCAN Unpack/1  "<HEV_Ctrl_PwtrCAN_Tx_0CFF2082>"
  PwtrCAN/1 -> Bus Selector2/1

== system CtrlStrct_VNT_Level1/VNT_Level_1_CAN/Body_Ctrl/BodyCtrl_VehCAN Tx ==
  note: Function of CAN transmit
      | ・conversion fromCAN application signal to signal of CAN message
  note: CAN transmit
  note: Body Control
  BodyCtrl_VehCAN_Tx_Apli : Inport
  BodyCtrl_VehCAN Pack : canmsglib/CAN Pack  CANdbFile=HEV_CANDB.dbc  MsgList=BodyCtrl_VehCAN_Tx  MsgName=BodyCtrl_VehCAN_Tx  MsgIDType=Extended (29-bit identifier)  MsgIdentifier=218079272  MsgLength=8  SignalInfo=BdyCtrl_Door_open_flag$1$1$1$2$1$0$1$0$0$1$#BdyCtrl_Engine_hood_open_flag$1$1$1$2$1$0$1$0$0$1$#BdyCtrl_Idlestop_cancel$0$1$1$2$1$0$1$0$0$1$#  NSignals=3  StartBits=str2num('[int32(1);int32(1);int32(0)]')  SignalSizes=str2num('[int32(1);int32(1);int32(1)]')  ByteOrders=str2num('[int32(1);int32(1);int32(1)]')  DataTypes=str2num('[int32(2);int32(2);int32(2)]')  MultiplexTypes=str2num('[int32(1);int32(1);int32(1)]')  MultiplexValues=str2num('[double(0);double(0);double(0)]')  Factors=str2num('[double(1);double(1);double(1)]')  Offsets=str2num('[double(0);double(0);double(0)]')  Minimums=str2num('[double(0);double(0);double(0)]')  Maximums=str2num('[double(1);double(1);double(1)]')  Remote=off  ApplyMinMax=off  BusOutput=off
      settings: AttributesFormatString=<CANdbFile = %<CANdbFile>>  SourceProductName=Simulink Real-Time  SourceProductBaseCode=XP  DataFormat=CANdb specified signals
  Bus Creator1 : BusCreator  Inputs=1
  Bus Selector2 : BusSelector  OutputSignals=BdyCtrl_Idlestop_cancel,BdyCtrl_Engine_hood_open_flag,BdyCtrl_Door_open_flag
  BodyCtrl_VehCAN_Tx : Outport
  wires:
  Bus Selector2/1 -> BodyCtrl_VehCAN Pack/1  "<BdyCtrl_Idlestop_cancel>"
  Bus Selector2/2 -> BodyCtrl_VehCAN Pack/2  "<BdyCtrl_Engine_hood_open_flag>"
  Bus Creator1/1 -> BodyCtrl_VehCAN_Tx/1  "BodyCtrl_VehCAN_Tx"
  Bus Selector2/3 -> BodyCtrl_VehCAN Pack/3  "<BdyCtrl_Door_open_flag>"
  BodyCtrl_VehCAN Pack/1 -> Bus Creator1/1  "BodyCtrl_VehCAN_Tx_0CFFA028"
  BodyCtrl_VehCAN_Tx_Apli/1 -> Bus Selector2/1

== system CtrlStrct_VNT_Level1/VNT_Level_1_CAN/Body_Ctrl/BodyCtrl_VehCAN_Rx ==
  note: CAN receive
  note: Body Control
  note: Function of CAN receive
      | ・CAN message selection
      | ・conversion from CAN signal to CAN application signal with bus object
  VehCAN : Inport
  BodyCtrl_VehCAN Unpack : canmsglib/CAN Unpack  CANdbFile=HEV_CANDB.dbc  MsgList=BrakeCtrl_VehCAN_Tx  MsgName=BrakeCtrl_VehCAN_Tx  MsgIDType=Extended (29-bit identifier)  MsgIdentifier=218062859  MsgLength=8  SignalInfo=BrkCtrl_Regen_brake_torque_reque$16$16$1$1$1$0$1.000000e-02$0$-300$300$#BrkCtrl_Vehicle_speed$0$16$1$2$1$0$1.000000e-01$0$0$180$#  NSignals=2  IDPort=off  TimestampPort=off  ErrorPort=off  RemotePort=off  LengthPort=off  StatusPort=off  StartBits=str2num('[int32(16);int32(0)]')  SignalSizes=str2num('[int32(16);int32(16)]')  ByteOrders=str2num('[int32(1);int32(1)]')  DataTypes=str2num('[int32(1);int32(2)]')  MultiplexTypes=str2num('[int32(1);int32(1)]')  MultiplexValues=str2num('[double(0);double(0)]')  Factors=str2num('[double(1.000000e-02);double(1.000000e-01)]')  Offsets=str2num('[double(0);double(0)]')  Minimums=str2num('[double(-300);double(0)]')  Maximums=str2num('[double(300);double(180)]')  ApplyMinMax=off
      settings: AttributesFormatString=<CANdbFile = %<CANdbFile>>  SourceProductName=Simulink Real-Time  SourceProductBaseCode=XP  DataFormat=CANdb specified signals
  BodyCtrl_VehCAN Unpack2 : canmsglib/CAN Unpack  CANdbFile=HEV_CANDB.dbc  MsgList=Gateway_VehCAN_Tx_2  MsgName=Gateway_VehCAN_Tx_2  MsgIDType=Extended (29-bit identifier)  MsgIdentifier=218087813  MsgLength=8  SignalInfo=EngCtrl_Engine_speed_G$0$16$1$2$1$0$1.250000e-01$0$0$8192$#HEV_IdleStopCtrl_preparation_r_G$24$1$1$2$1$0$1$0$0$1$#HEV_IdleStopCtrl_request_G$25$1$1$2$1$0$1$0$0$1$#HEV_IdleStopCtrl_status_G$26$1$1$2$1$0$1$0$0$1$#TmCtrl_Gear_position_G$16$8$1$2$1$0$1$0$0$5$#  NSignals=5  IDPort=off  TimestampPort=off  ErrorPort=off  RemotePort=off  LengthPort=off  StatusPort=off  StartBits=str2num('[int32(0);int32(24);int32(25);int32(26);int32(16)]')  SignalSizes=str2num('[int32(16);int32(1);int32(1);int32(1);int32(8)]')  ByteOrders=str2num('[int32(1);int32(1);int32(1);int32(1);int32(1)]')  DataTypes=str2num('[int32(2);int32(2);int32(2);int32(2);int32(2)]')  MultiplexTypes=str2num('[int32(1);int32(1);int32(1);int32(1);int32(1)]')  MultiplexValues=str2num('[double(0);double(0);double(0);double(0);double(0)]')  Factors=str2num('[double(1.250000e-01);double(1);double(1);double(1);double(1)]')  Offsets=str2num('[double(0);double(0);double(0);double(0);double(0)]')  Minimums=str2num('[double(0);double(0);double(0);double(0);double(0)]')  Maximums=str2num('[double(8192);double(1);double(1);double(1);double(5)]')  ApplyMinMax=off
      settings: AttributesFormatString=<CANdbFile = %<CANdbFile>>  SourceProductName=Simulink Real-Time  SourceProductBaseCode=XP  DataFormat=CANdb specified signals
  Bus Creator : BusCreator  Inputs=3
  Bus Selector4 : BusSelector  OutputSignals=Gateway_VehCAN_Tx_0CFFC185
  Bus Selector7 : BusSelector  OutputSignals=BrakeCtrl_VehCAN_Tx_0CFF600B
  Rate Transition1 : RateTransition  Deterministic=off
      settings: AttributesFormatString=<Deterministic=%<Deterministic>>
  Terminator{3..6} (4 alike) : Terminator
  BodyCtrl_VehCAN_Rx : Outport
  wires:
  BodyCtrl_VehCAN Unpack2/2 -> Terminator3/1
  Bus Selector7/1 -> BodyCtrl_VehCAN Unpack/1  "<BrakeCtrl_VehCAN_Tx_0CFF600B>"
  BodyCtrl_VehCAN Unpack/2 -> Bus Creator/1  "BrkCtrl_Vehicle_speed"
  BodyCtrl_VehCAN Unpack2/3 -> Terminator5/1
  BodyCtrl_VehCAN Unpack/1 -> Terminator4/1  "BrkCtrl_Regen_brake_torque_request"
  VehCAN/1 -> Bus Selector4/1, Bus Selector7/1
  BodyCtrl_VehCAN Unpack2/4 -> Bus Creator/3  "HEVCtrl_IdleStop_status"
  Bus Selector4/1 -> BodyCtrl_VehCAN Unpack2/1  "<Gateway_VehCAN_Tx_0CFFC185>"
  BodyCtrl_VehCAN Unpack2/1 -> Bus Creator/2  "EngCtrl_Engine_speed"
  BodyCtrl_VehCAN Unpack2/5 -> Terminator6/1
  Bus Creator/1 -> Rate Transition1/1
  Rate Transition1/1 -> BodyCtrl_VehCAN_Rx/1  "BodyCtrl_VehCAN_Rx"

== system CtrlStrct_VNT_Level1/VNT_Level_1_CAN/Brake_Ctrl/BrakeCtrl_VehCAN Tx ==
  note: CAN transmit
  note: Brake Control
  note: Function of CAN transmit
      | ・conversion fromCAN application signal to signal of CAN message
  BrakeCtrl_VehCAN_Tx_Apli : Inport
  BrakeCtrl_VehCAN Pack : canmsglib/CAN Pack  CANdbFile=HEV_CANDB.dbc  MsgList=BrakeCtrl_VehCAN_Tx  MsgName=BrakeCtrl_VehCAN_Tx  MsgIDType=Extended (29-bit identifier)  MsgIdentifier=218062859  MsgLength=8  SignalInfo=BrkCtrl_Regen_brake_torque_reque$16$16$1$1$1$0$1.000000e-02$0$-300$300$#BrkCtrl_Vehicle_speed$0$16$1$2$1$0$1.000000e-01$0$0$180$#  NSignals=2  StartBits=str2num('[int32(16);int32(0)]')  SignalSizes=str2num('[int32(16);int32(16)]')  ByteOrders=str2num('[int32(1);int32(1)]')  DataTypes=str2num('[int32(1);int32(2)]')  MultiplexTypes=str2num('[int32(1);int32(1)]')  MultiplexValues=str2num('[double(0);double(0)]')  Factors=str2num('[double(1.000000e-02);double(1.000000e-01)]')  Offsets=str2num('[double(0);double(0)]')  Minimums=str2num('[double(-300);double(0)]')  Maximums=str2num('[double(300);double(180)]')  Remote=off  ApplyMinMax=off  BusOutput=off
      settings: AttributesFormatString=<CANdbFile = %<CANdbFile>>  SourceProductName=Simulink Real-Time  SourceProductBaseCode=XP  DataFormat=CANdb specified signals
  Bus Creator1 : BusCreator  Inputs=1
  Bus Selector4 : BusSelector  OutputSignals=BrkCtrl_Regen_brake_torque_request,BrkCtrl_Vehicle_speed
  BrakeCtrl_VehCAN_Tx : Outport
  wires:
  Bus Selector4/2 -> BrakeCtrl_VehCAN Pack/2  "<BrkCtrl_Vehicle_speed>"
  BrakeCtrl_VehCAN_Tx_Apli/1 -> Bus Selector4/1
  Bus Creator1/1 -> BrakeCtrl_VehCAN_Tx/1  "BrakeCtrl_VehCAN_Tx"
  Bus Selector4/1 -> BrakeCtrl_VehCAN Pack/1  "<BrkCtrl_Regen_brake_torque_request>"
  BrakeCtrl_VehCAN Pack/1 -> Bus Creator1/1  "BrakeCtrl_VehCAN_Tx_0CFF600B"
